simulink model "Pole_Placement_mit_zustandsregler"  (Simulink 7.5)
settings: Solver=ode45  StartTime=0.0  StopTime=10.0  RelTol=1e-3
values from neighbouring files (symbols this model uses):
  KV = KV'    [Reglerauslegung.m]    (also in Test_Reglerauslegung.m; auslegung.m)
undefined symbols (not defined in the file or in its folder): A, b, cT
settings Model: Creator=Mattse  LastModifiedBy=Mattse

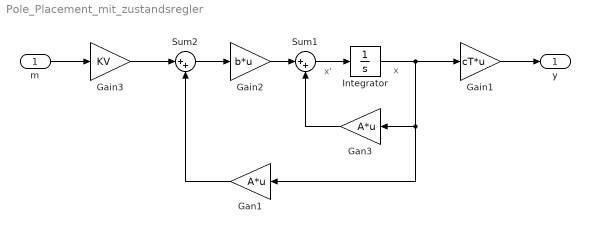
== system Pole_Placement_mit_zustandsregler ==
  note: x'
  note: x
  m : Inport  OutDataType=fixdt(1, 16)  OutScaling=2^0
  Gain1 : Gain  Gain=cT*u  ParameterDataType=fixdt(1, 16)  ParameterScaling=2^0  OutDataType=fixdt(1, 16)  OutScaling=2^0
  Gain2 : Gain  Gain=b*u  ParameterDataType=fixdt(1, 16)  ParameterScaling=2^0  OutDataType=fixdt(1, 16)  OutScaling=2^0
  Gain3 : Gain  Gain=KV  ParameterDataType=fixdt(1, 16)  ParameterScaling=2^0  OutDataType=fixdt(1, 16)  OutScaling=2^0
  Gan1 : Gain  Gain=A*u  ParameterDataType=fixdt(1, 16)  ParameterScaling=2^0  OutDataType=fixdt(1, 16)  OutScaling=2^0
  Gan3 : Gain  Gain=A*u  ParameterDataType=fixdt(1, 16)  ParameterScaling=2^0  OutDataType=fixdt(1, 16)  OutScaling=2^0
  Integrator : Integrator
  Sum1 : Sum  Inputs=|++  OutDataType=fixdt(1, 16)  OutScaling=2^0
  Sum2 : Sum  Inputs=|++  OutDataType=fixdt(1, 16)  OutScaling=2^0
  y : Outport  OutDataType=fixdt(1, 16)  OutScaling=2^0
  wires:
  Integrator/1 -> Gain1/1, Gan3/1, Gan1/1
  Sum1/1 -> Integrator/1
  Gain2/1 -> Sum1/1
  Gan3/1 -> Sum1/2
  Gain1/1 -> y/1
  Gan1/1 -> Sum2/2
  Sum2/1 -> Gain2/1
  m/1 -> Gain3/1
  Gain3/1 -> Sum2/1
